simulink model "nn_ruido"  (R2023a)
settings: Solver=VariableStepAuto  StartTime=0.0  StopTime=1000  RelTol=1e-3
values from neighbouring files (symbols this model uses):
  A = 0.0154    [parametros.m]    (also in variables.mat)
  az1 = 1    [parametros.m]    (also in variables.mat)
  az2 = 1    [parametros.m]    (also in variables.mat)
  az3 = 1    [parametros.m]    (also in variables.mat)
  g = 9.8    [parametros.m]    (also in variables.mat)
  H_star1 = 0.4    [parametros.m]    (also in variables.mat)
  H_star2 = 0.15    [parametros.m]    (also in variables.mat)
  Sn = 5e-5    (= 5e-05)    [parametros.m]    (also in variables.mat)
settings Model: Creator=empg0  LastModifiedBy=empg0

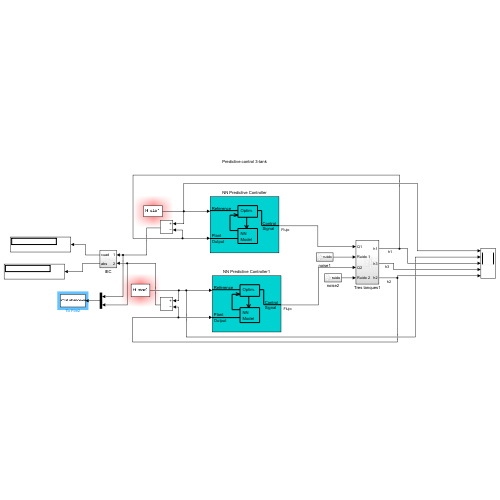
[thumbnail: Simulink's stored preview of the top-level diagram]
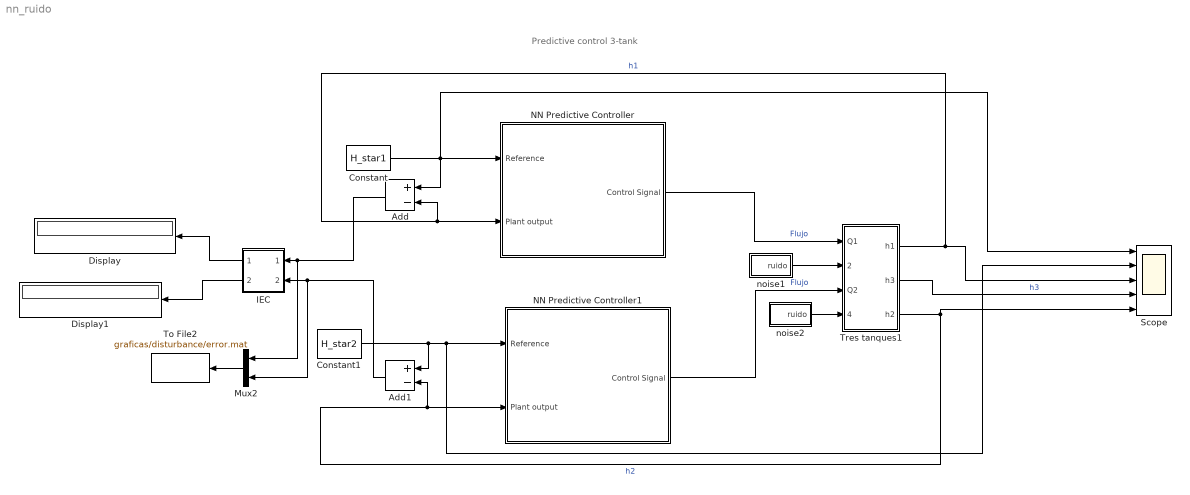
== system nn_ruido ==
  note: Predictive control 3-tank
  Add : Sum  Inputs=+-
  Add1 : Sum  Inputs=+-
  Constant : Constant  Value=H_star1
  Constant1 : Constant  Value=H_star2
  Display : Display
  Display1 : Display
  IEC : Subsystem
  Mux2 : Mux  Inputs=2
  NN Predictive Controller : Subsystem  mask(NN Predictive Controller){N2=7, Nu=2, Ts=0.5, rho=0.05, alpha=0.001, csrchfun=csrchbac, maxiter=2, S1=7, Ni=2, Nj=2, sim_file=planta, trainfun=trainlm, Use_validation=1, Use_Testing=0, max_i=0.1, min_i=0, sam_training=8000, epochs=200, minp=0.00083750919477898130849, maxp=0.099220790480832016245, mint=0, maxt=0.099220790480832016245, Normalize=0, IW=[-20.531676995171057598 18.704335179754611573;0.00020386653261894715898 -0.00065105597203892015979;0.11039206030581787121 0.078287285196172784474;-4.2899902912608469663 -2.5279624927180339711;-7.6432027343615454029 11.5285765668885265;-0.017993776662611957878 0.0088727669270464385592;-9.0344400995814524435 3.9540417662274571775], LW1_2=[14.923957143723018959 -17.978284009820111322;-0.71975082637667153751 0.32012412094941411489;0.64966823503412085561 0.085723391515673319496;55.495721009703864013 -51.282194417149113974;-3.6640121805562331225 2.3449172788885150887;-0.52558872900568831543 0.055226005018602114527;-1.7503201452350198863 4.144472061218764658], LW2_1=[-2.1959814678618032602 -3.2437397056361580994 7.2781964126742613175 2.1984051114526992343 1.7353616977917190045 -2.0712307468921604681 2.1983321974786087516], B1=[18.564420214207171256;9.6247423275479970783;-3.5269187756800972622;-67.658376524939384922;-4.4107470426168395861;0.061944283876979457093;-40.321949269656272463], B2=18.964938123059841502, max_i_int=20, min_i_int=5, limit_output=1, max_output=0.62, min_output=0, Use_Previous_Weights=1}
      mask prompts: Ts "Sample time"; rho "rho (typically = 0.03)"; alpha "alpha (typically = 0.001)"; csrchfun "Minimization rutine"; trainfun "Training function"
      mask help: NN Predictive Controller. You first train a neural network model of the plant to be controlled. The controller uses the plant model to predict plant performance over a specified time horizon. An optimization algorithm determines the control signal that optimizes plant performance over this horizon. Double click the NN Predictive Controller block to train the plant model and set the controller parameters.
      mask init:
      | xl = [0   .53   .53     .85   .85  .53  .53  NaN .85  .92 .92];
      | yl = [.95 .95 1.05  1.05   .82  .82  .95  NaN  .95 .95 .65];
      | x2 = [0 .53    NaN .92 1.2 NaN .53 .85 .85 .53 .53 ];
      | y2 = [.39 .39   NaN .65 .65 NaN .59 .59 .29 .29  .59];
      | x3 = [.67 .67 NaN .64 .67 .70 NaN .53 .4   .4   .53 NaN .46 .53 .46];
      | y3 = [.59 .82 NaN .66 .59 .66 NaN .55 .55 .86 .86 NaN  .89 .86 .83];
      | 
      | x1t=.03; y1t=.31;
      | x2t=.03; y2t=.8;
      | x8t=.03;y8t=.21;
      | x3t=.77; y3t=.53;
      | x4t=.77; y4t=.44;
      | x5t=.45; y5t=.76;
      | x6t=.45; y6t=.35;
      | x7t=.45; y7t=.25;
      settings: OpenFcn=nncontrolutil('nnpredict','',gcbh,gcb);
      mask TypeOptions csrchfun: csrchgol | csrchbac | csrchhyb | csrchbre | csrchcha
      mask TypeOptions trainfun: trainbfg | trainbr  | traincgb | traincgf | traincgp | traingd | traingdm | traingda | traingdx | trainlm  | trainoss | trainrp  | trainscg
      mask Display:
      | plot([[xl NaN x2]*.9-.075 ], [[yl  NaN y2]*.9-.1 ]);
      | plot([[x3]*.9-.075 ], [[y3]*.9-.1 ]);
      | text(x1t,y1t,'Plant');
      | text(x8t,y8t,'Output');
      | text(x2t,y2t,'Reference');
      | text(x3t,y3t,'Control');
      | text(x4t,y4t,'Signal');
      | text(x5t,y5t,'Optim.');
      | text(x6t,y6t,'NN');
      | text(x7t,y7t,'Model');
  NN Predictive Controller1 : Subsystem  mask(NN Predictive Controller){N2=7, Nu=2, Ts=0.5, rho=0.05, alpha=0.001, csrchfun=csrchbac, maxiter=2, S1=7, Ni=2, Nj=2, sim_file=planta, trainfun=trainlm, Use_validation=1, Use_Testing=0, max_i=0.1, min_i=0, sam_training=8000, epochs=200, minp=0.00083750919477898130849, maxp=0.099220790480832016245, mint=0, maxt=0.099220790480832016245, Normalize=0, IW=[-20.531676995171057598 18.704335179754611573;0.00020386653261894715898 -0.00065105597203892015979;0.11039206030581787121 0.078287285196172784474;-4.2899902912608469663 -2.5279624927180339711;-7.6432027343615454029 11.5285765668885265;-0.017993776662611957878 0.0088727669270464385592;-9.0344400995814524435 3.9540417662274571775], LW1_2=[14.923957143723018959 -17.978284009820111322;-0.71975082637667153751 0.32012412094941411489;0.64966823503412085561 0.085723391515673319496;55.495721009703864013 -51.282194417149113974;-3.6640121805562331225 2.3449172788885150887;-0.52558872900568831543 0.055226005018602114527;-1.7503201452350198863 4.144472061218764658], LW2_1=[-2.1959814678618032602 -3.2437397056361580994 7.2781964126742613175 2.1984051114526992343 1.7353616977917190045 -2.0712307468921604681 2.1983321974786087516], B1=[18.564420214207171256;9.6247423275479970783;-3.5269187756800972622;-67.658376524939384922;-4.4107470426168395861;0.061944283876979457093;-40.321949269656272463], B2=18.964938123059841502, max_i_int=20, min_i_int=5, limit_output=1, max_output=0.62, min_output=0, Use_Previous_Weights=1}
      mask prompts: Ts "Sample time"; rho "rho (typically = 0.03)"; alpha "alpha (typically = 0.001)"; csrchfun "Minimization rutine"; trainfun "Training function"
      mask help: NN Predictive Controller. You first train a neural network model of the plant to be controlled. The controller uses the plant model to predict plant performance over a specified time horizon. An optimization algorithm determines the control signal that optimizes plant performance over this horizon. Double click the NN Predictive Controller block to train the plant model and set the controller parameters.
      mask init: same as nn_ruido/NN Predictive Controller
      settings: OpenFcn=nncontrolutil('nnpredict','',gcbh,gcb);
      mask TypeOptions csrchfun: csrchgol | csrchbac | csrchhyb | csrchbre | csrchcha
      mask TypeOptions trainfun: trainbfg | trainbr  | traincgb | traincgf | traincgp | traingd | traingdm | traingda | traingdx | trainlm  | trainoss | trainrp  | trainscg
      mask Display:
      | plot([[xl NaN x2]*.9-.075 ], [[yl  NaN y2]*.9-.1 ]);
      | plot([[x3]*.9-.075 ], [[y3]*.9-.1 ]);
      | text(x1t,y1t,'Plant');
      | text(x8t,y8t,'Output');
      | text(x2t,y2t,'Reference');
      | text(x3t,y3t,'Control');
      | text(x4t,y4t,'Signal');
      | text(x5t,y5t,'Optim.');
      | text(x6t,y6t,'NN');
      | text(x7t,y7t,'Model');
  Scope : Scope  NumInputPorts=5
  To File2 : ToFile  Filename=graficas/disturbance/error.mat  MatrixName=error  SampleTime=0.5
  Tres tanques1 : Subsystem
  noise1 : Subsystem
  noise2 : Subsystem
  wires:
  NN Predictive Controller/1(Control Signal) -> Tres tanques1/1(Q1)  "Flujo"
  NN Predictive Controller1/1(Control Signal) -> Tres tanques1/3(Q2)  "Flujo"
  Tres tanques1/1(h1) -> Add/2, NN Predictive Controller/2(Plant output), Scope/3  "h1"
  Constant/1 -> Add/1, Scope/1, NN Predictive Controller/1(Reference)
  Constant1/1 -> Add1/1, Scope/2, NN Predictive Controller1/1(Reference)
  Tres tanques1/3(h2) -> Add1/2, NN Predictive Controller1/2(Plant output), Scope/5  "h2"
  Tres tanques1/2(h3) -> Scope/4  "h3"
  Add/1 -> Mux2/1, IEC/1(In1)
  Add1/1 -> Mux2/2, IEC/2(In2)
  IEC/1(cuad) -> Display/1
  Mux2/1 -> To File2/1
  noise1/1(ruido) -> Tres tanques1/2(Ruido 1)
  noise2/1(ruido) -> Tres tanques1/4(Ruido 2)
  IEC/2(abs) -> Display1/1

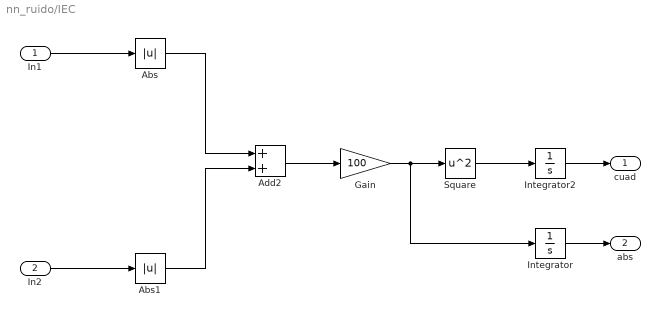
== system nn_ruido/IEC ==
  In1 : Inport
  In2 : Inport  Port=2
  Abs : Abs  SaturateOnIntegerOverflow=off
  Abs1 : Abs  SaturateOnIntegerOverflow=off
  Add2 : Sum
  Gain : Gain  Gain=100
  Integrator : Integrator
  Integrator2 : Integrator
  Square : Math  Operator=square
  cuad : Outport
  abs : Outport  Port=2
  wires:
  Abs1/1 -> Add2/2
  Abs/1 -> Add2/1
  In2/1 -> Abs1/1
  Square/1 -> Integrator2/1
  Integrator2/1 -> cuad/1
  In1/1 -> Abs/1
  Add2/1 -> Gain/1
  Gain/1 -> Integrator/1, Square/1
  Integrator/1 -> abs/1

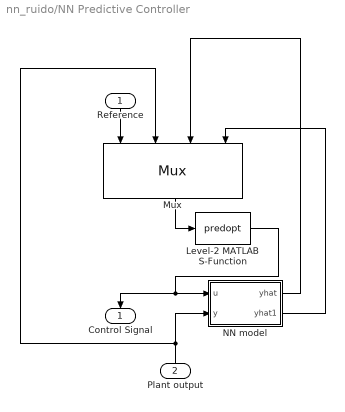
== system nn_ruido/NN Predictive Controller ==
  Reference : Inport
  Plant output : Inport  Port=2
  Level-2 MATLAB S-Function : M-S-Function  FunctionName=predopt  Parameters=N2,Ts,Nu,maxiter,csrchfun,rho,alpha,S1,IW,LW1_2,LW2_1,B1,B2,Ni,Nj,min_i,max_i,minp,maxp,mint,maxt,Normalize
  Mux : Mux
      settings: DisplayOption=signals
  NN model : Subsystem
  Control Signal : Outport
  wires:
  Mux/1 -> Level-2 MATLAB S-Function/1
  Level-2 MATLAB S-Function/1 -> NN model/1(u), Control Signal/1
  NN model/2(yhat1) -> Mux/4
  NN model/1(yhat) -> Mux/3
  Reference/1 -> Mux/1
  Plant output/1 -> NN model/2(y), Mux/2

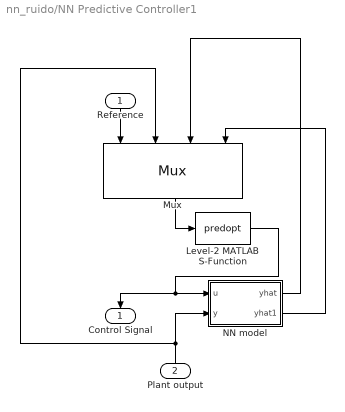
== system nn_ruido/NN Predictive Controller1 ==
  Reference : Inport
  Plant output : Inport  Port=2
  Level-2 MATLAB S-Function : M-S-Function  FunctionName=predopt  Parameters=N2,Ts,Nu,maxiter,csrchfun,rho,alpha,S1,IW,LW1_2,LW2_1,B1,B2,Ni,Nj,min_i,max_i,minp,maxp,mint,maxt,Normalize
  Mux : Mux
      settings: DisplayOption=signals
  NN model : Subsystem
  Control Signal : Outport
  wires:
  Mux/1 -> Level-2 MATLAB S-Function/1
  Level-2 MATLAB S-Function/1 -> NN model/1(u), Control Signal/1
  NN model/2(yhat1) -> Mux/4
  NN model/1(yhat) -> Mux/3
  Reference/1 -> Mux/1
  Plant output/1 -> NN model/2(y), Mux/2

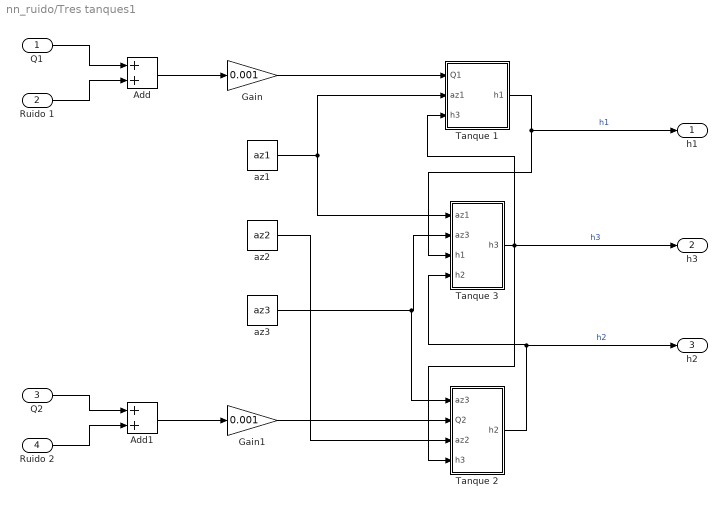
== system nn_ruido/Tres tanques1 ==
  Q1 : Inport
  Ruido 1 : Inport  Port=2
  Q2 : Inport  Port=3
  Ruido 2 : Inport  Port=4
  Add : Sum
  Add1 : Sum
  Gain : Gain  Gain=0.001
  Gain1 : Gain  Gain=0.001
  Tanque 1 : Subsystem
  Tanque 2 : Subsystem
  Tanque 3 : Subsystem
  az1 : Constant  Value=az1
  az2 : Constant  Value=az2
  az3 : Constant  Value=az3
  h1 : Outport
  h3 : Outport  Port=2
  h2 : Outport  Port=3
  wires:
  Tanque 2/1(h2) -> Tanque 3/4(h2), h2/1  "h2"
  Tanque 1/1(h1) -> Tanque 3/3(h1), h1/1  "h1"
  Gain1/1 -> Tanque 2/2(Q2)
  Tanque 3/1(h3) -> Tanque 2/4(h3), h3/1, Tanque 1/3(h3)  "h3"
  az3/1 -> Tanque 2/1(az3), Tanque 3/2(az3)
  az1/1 -> Tanque 3/1(az1), Tanque 1/2(az1)
  az2/1 -> Tanque 2/3(az2)
  Gain/1 -> Tanque 1/1(Q1)
  Add/1 -> Gain/1
  Q1/1 -> Add/1
  Ruido 1/1 -> Add/2
  Add1/1 -> Gain1/1
  Q2/1 -> Add1/1
  Ruido 2/1 -> Add1/2

== system nn_ruido/noise1 ==
  Constant : Constant  Value=0
  Manual Switch : ManualSwitch
  urn : UniformRandomNumber  Minimum=-0.1*0.1  Maximum=0.1*0.1  Seed=140  SampleTime=20
  ruido : Outport
  wires:
  urn/1 -> Manual Switch/1
  Constant/1 -> Manual Switch/2
  Manual Switch/1 -> ruido/1

== system nn_ruido/noise2 ==
  Constant : Constant  Value=0
  Manual Switch : ManualSwitch
  urn : UniformRandomNumber  Minimum=-0.1*0.1  Maximum=0.1*0.1  Seed=150  SampleTime=20
  ruido : Outport
  wires:
  urn/1 -> Manual Switch/1
  Constant/1 -> Manual Switch/2
  Manual Switch/1 -> ruido/1

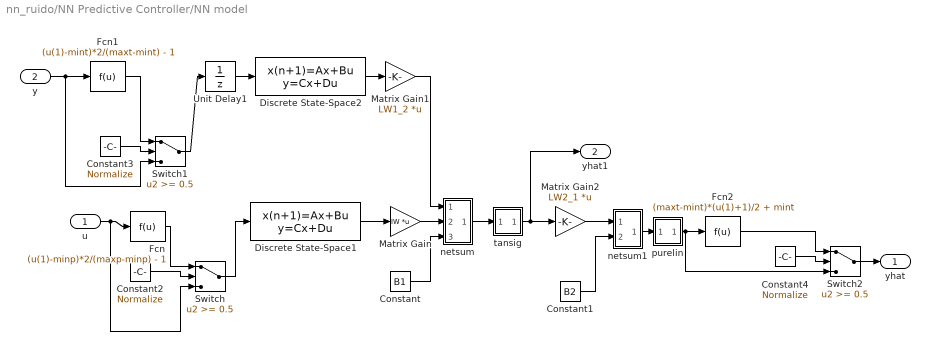
== system nn_ruido/NN Predictive Controller/NN model ==
  u : Inport
  y : Inport  Port=2
  Constant : Constant  Value=B1
  Constant1 : Constant  Value=B2
  Constant2 : Constant  Value=Normalize
  Constant3 : Constant  Value=Normalize
  Constant4 : Constant  Value=Normalize
  Discrete State-Space1 : DiscreteStateSpace  A=[0 zeros(1,Ni-2);eye(Ni-2,Ni-1)]  B=[zeros(double(Ni==1));eye(Ni-1,1)]  C=[0 zeros(1,Ni-2);eye(Ni-1,Ni-1)]  D=eye(Ni,1)  SampleTime=Ts
  Discrete State-Space2 : DiscreteStateSpace  A=[0 zeros(1,Nj-2);eye(Nj-2,Nj-1)]  B=[zeros(double(Nj==1));eye(Nj-1,1)]  C=[0 zeros(1,Nj-2);eye(Nj-1,Nj-1)]  D=eye(Nj,1)  SampleTime=Ts
  Fcn : Fcn  Expr=(u(1)-minp)*2/(maxp-minp) - 1
  Fcn1 : Fcn  Expr=(u(1)-mint)*2/(maxt-mint) - 1
  Fcn2 : Fcn  Expr=(maxt-mint)*(u(1)+1)/2 + mint
  Matrix Gain : Gain  Gain=IW  Multiplication=Matrix(K*u)  SaturateOnIntegerOverflow=on  OutDataTypeStr=Inherit: Same as input  ParamDataTypeStr=Inherit: Same as input
  Matrix Gain1 : Gain  Gain=LW1_2  Multiplication=Matrix(K*u)  SaturateOnIntegerOverflow=on  OutDataTypeStr=Inherit: Same as input  ParamDataTypeStr=Inherit: Same as input
  Matrix Gain2 : Gain  Gain=LW2_1  Multiplication=Matrix(K*u)  SaturateOnIntegerOverflow=on  OutDataTypeStr=Inherit: Same as input  ParamDataTypeStr=Inherit: Same as input
  Switch : Switch  Threshold=0.5  ZeroCross=off
  Switch1 : Switch  Threshold=0.5  ZeroCross=off
  Switch2 : Switch  Threshold=0.5  ZeroCross=off
  Unit Delay1 : UnitDelay  SampleTime=Ts  HasFrameUpgradeWarning=on
  netsum : Subsystem
      mask Display: disp('+')
  netsum1 : Subsystem
      mask Display: disp('+')
  purelin : Subsystem
      mask Display: plot([-1 1],[0 0],[-1 1],[-1 1])
  tansig : Subsystem
      mask Display: plot([-1 1],[0 0],[-1 -.9 -.8 -.7 -.6 -.5 -.4 -.3 -.2 -.1 0 .1 .2 .3 .4 .5 .6 .7 .8 .9 1],2./(1+exp(-8*[-1 -.9 -.8 -.7 -.6 -.5 -.4 -.3 -.2 -.1 0 .1 .2 .3 .4 .5 .6 .7 .8 .9 1]))-1)
  yhat : Outport
  yhat1 : Outport  Port=2
  wires:
  netsum1/1(Out1) -> purelin/1(n)
  Constant1/1 -> netsum1/2(In2)
  Matrix Gain2/1 -> netsum1/1(In1)
  netsum/1(Out1) -> tansig/1(n)
  Constant/1 -> netsum/3(In3)
  Matrix Gain1/1 -> netsum/1(In1)
  Matrix Gain/1 -> netsum/2(In2)
  tansig/1(a) -> Matrix Gain2/1, yhat1/1
  Discrete State-Space1/1 -> Matrix Gain/1
  Fcn/1 -> Switch/1
  Switch/1 -> Discrete State-Space1/1
  u/1 -> Fcn/1, Switch/3
  Constant2/1 -> Switch/2
  Discrete State-Space2/1 -> Matrix Gain1/1
  Unit Delay1/1 -> Discrete State-Space2/1
  Constant3/1 -> Switch1/2
  Switch1/1 -> Unit Delay1/1
  Fcn1/1 -> Switch1/1
  y/1 -> Fcn1/1, Switch1/3
  Constant4/1 -> Switch2/2
  Switch2/1 -> yhat/1
  Fcn2/1 -> Switch2/1
  purelin/1(a) -> Fcn2/1, Switch2/3

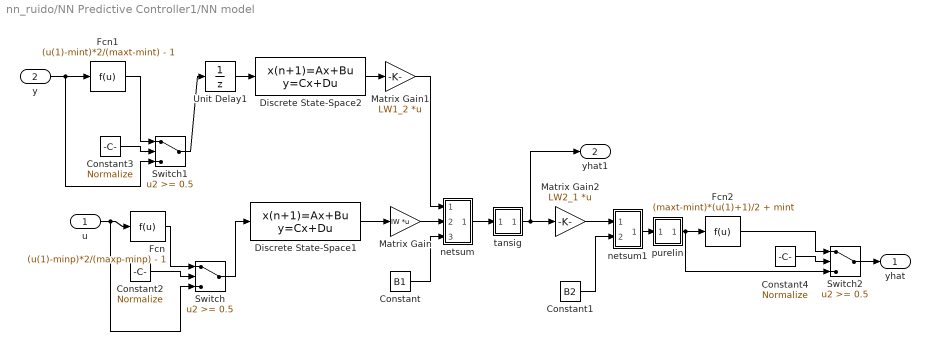
== system nn_ruido/NN Predictive Controller1/NN model ==
  u : Inport
  y : Inport  Port=2
  Constant : Constant  Value=B1
  Constant1 : Constant  Value=B2
  Constant2 : Constant  Value=Normalize
  Constant3 : Constant  Value=Normalize
  Constant4 : Constant  Value=Normalize
  Discrete State-Space1 : DiscreteStateSpace  A=[0 zeros(1,Ni-2);eye(Ni-2,Ni-1)]  B=[zeros(double(Ni==1));eye(Ni-1,1)]  C=[0 zeros(1,Ni-2);eye(Ni-1,Ni-1)]  D=eye(Ni,1)  SampleTime=Ts
  Discrete State-Space2 : DiscreteStateSpace  A=[0 zeros(1,Nj-2);eye(Nj-2,Nj-1)]  B=[zeros(double(Nj==1));eye(Nj-1,1)]  C=[0 zeros(1,Nj-2);eye(Nj-1,Nj-1)]  D=eye(Nj,1)  SampleTime=Ts
  Fcn : Fcn  Expr=(u(1)-minp)*2/(maxp-minp) - 1
  Fcn1 : Fcn  Expr=(u(1)-mint)*2/(maxt-mint) - 1
  Fcn2 : Fcn  Expr=(maxt-mint)*(u(1)+1)/2 + mint
  Matrix Gain : Gain  Gain=IW  Multiplication=Matrix(K*u)  SaturateOnIntegerOverflow=on  OutDataTypeStr=Inherit: Same as input  ParamDataTypeStr=Inherit: Same as input
  Matrix Gain1 : Gain  Gain=LW1_2  Multiplication=Matrix(K*u)  SaturateOnIntegerOverflow=on  OutDataTypeStr=Inherit: Same as input  ParamDataTypeStr=Inherit: Same as input
  Matrix Gain2 : Gain  Gain=LW2_1  Multiplication=Matrix(K*u)  SaturateOnIntegerOverflow=on  OutDataTypeStr=Inherit: Same as input  ParamDataTypeStr=Inherit: Same as input
  Switch : Switch  Threshold=0.5  ZeroCross=off
  Switch1 : Switch  Threshold=0.5  ZeroCross=off
  Switch2 : Switch  Threshold=0.5  ZeroCross=off
  Unit Delay1 : UnitDelay  SampleTime=Ts  HasFrameUpgradeWarning=on
  netsum : Subsystem
      mask Display: disp('+')
  netsum1 : Subsystem
      mask Display: disp('+')
  purelin : Subsystem
      mask Display: plot([-1 1],[0 0],[-1 1],[-1 1])
  tansig : Subsystem
      mask Display: plot([-1 1],[0 0],[-1 -.9 -.8 -.7 -.6 -.5 -.4 -.3 -.2 -.1 0 .1 .2 .3 .4 .5 .6 .7 .8 .9 1],2./(1+exp(-8*[-1 -.9 -.8 -.7 -.6 -.5 -.4 -.3 -.2 -.1 0 .1 .2 .3 .4 .5 .6 .7 .8 .9 1]))-1)
  yhat : Outport
  yhat1 : Outport  Port=2
  wires:
  netsum1/1(Out1) -> purelin/1(n)
  Constant1/1 -> netsum1/2(In2)
  Matrix Gain2/1 -> netsum1/1(In1)
  netsum/1(Out1) -> tansig/1(n)
  Constant/1 -> netsum/3(In3)
  Matrix Gain1/1 -> netsum/1(In1)
  Matrix Gain/1 -> netsum/2(In2)
  tansig/1(a) -> Matrix Gain2/1, yhat1/1
  Discrete State-Space1/1 -> Matrix Gain/1
  Fcn/1 -> Switch/1
  Switch/1 -> Discrete State-Space1/1
  u/1 -> Fcn/1, Switch/3
  Constant2/1 -> Switch/2
  Discrete State-Space2/1 -> Matrix Gain1/1
  Unit Delay1/1 -> Discrete State-Space2/1
  Constant3/1 -> Switch1/2
  Switch1/1 -> Unit Delay1/1
  Fcn1/1 -> Switch1/1
  y/1 -> Fcn1/1, Switch1/3
  Constant4/1 -> Switch2/2
  Switch2/1 -> yhat/1
  Fcn2/1 -> Switch2/1
  purelin/1(a) -> Fcn2/1, Switch2/3

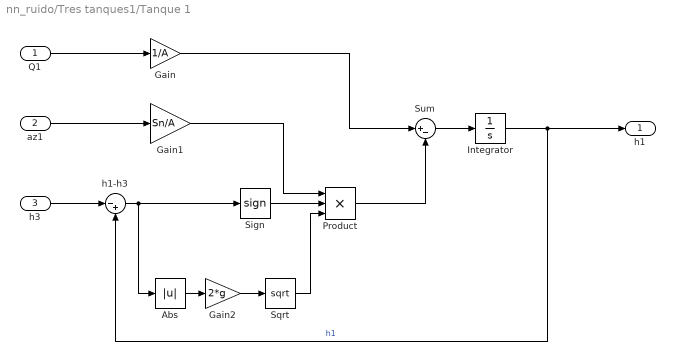
== system nn_ruido/Tres tanques1/Tanque 1 ==
  Q1 : Inport
  az1 : Inport  Port=2
  h3 : Inport  Port=3
  Abs : Abs  SaturateOnIntegerOverflow=off
  Gain : Gain  Gain=1/A
  Gain1 : Gain  Gain=Sn/A
  Gain2 : Gain  Gain=2*g
  Integrator : Integrator  LimitOutput=on  UpperSaturationLimit=0.62  LowerSaturationLimit=0
  Product : Product  Inputs=3
  Sign : Signum
  Sqrt : Sqrt
  Sum : Sum  Inputs=|+-
  h1-h3 : Sum  Inputs=|-+
  h1 : Outport
  wires:
  h3/1 -> h1-h3/1
  Sum/1 -> Integrator/1
  Gain2/1 -> Sqrt/1
  Gain1/1 -> Product/1
  Sqrt/1 -> Product/3
  Sign/1 -> Product/2
  h1-h3/1 -> Abs/1, Sign/1
  Q1/1 -> Gain/1
  az1/1 -> Gain1/1
  Integrator/1 -> h1/1, h1-h3/2  "h1"
  Product/1 -> Sum/2
  Gain/1 -> Sum/1
  Abs/1 -> Gain2/1

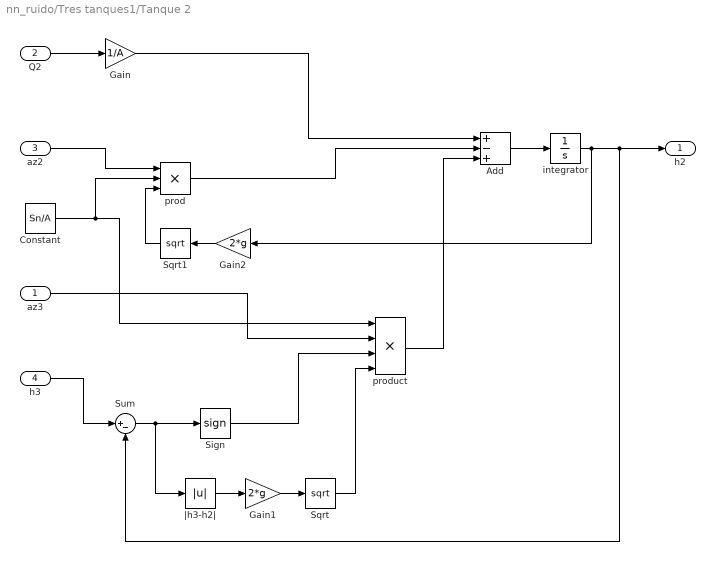
== system nn_ruido/Tres tanques1/Tanque 2 ==
  az3 : Inport
  Q2 : Inport  Port=2
  az2 : Inport  Port=3
  h3 : Inport  Port=4
  Add : Sum  Inputs=+-+
  Constant : Constant  Value=Sn/A
  Gain : Gain  Gain=1/A
  Gain1 : Gain  Gain=2*g
  Gain2 : Gain  Gain=2*g
  Sign : Signum
  Sqrt : Sqrt
  Sqrt1 : Sqrt
  Sum : Sum  Inputs=|+-
  integrator : Integrator  LimitOutput=on  UpperSaturationLimit=0.62  LowerSaturationLimit=0
  prod : Product  Inputs=3
  product : Product  Inputs=4
  |h3-h2| : Abs  SaturateOnIntegerOverflow=off
  h2 : Outport
  wires:
  |h3-h2|/1 -> Gain1/1
  prod/1 -> Add/2
  product/1 -> Add/3
  Add/1 -> integrator/1
  Gain/1 -> Add/1
  Constant/1 -> product/1, prod/2
  Gain1/1 -> Sqrt/1
  Sum/1 -> |h3-h2|/1, Sign/1
  az2/1 -> prod/1
  az3/1 -> product/2
  Sqrt1/1 -> prod/3
  Sqrt/1 -> product/4
  Sign/1 -> product/3
  h3/1 -> Sum/1
  integrator/1 -> Gain2/1, h2/1, Sum/2
  Gain2/1 -> Sqrt1/1
  Q2/1 -> Gain/1

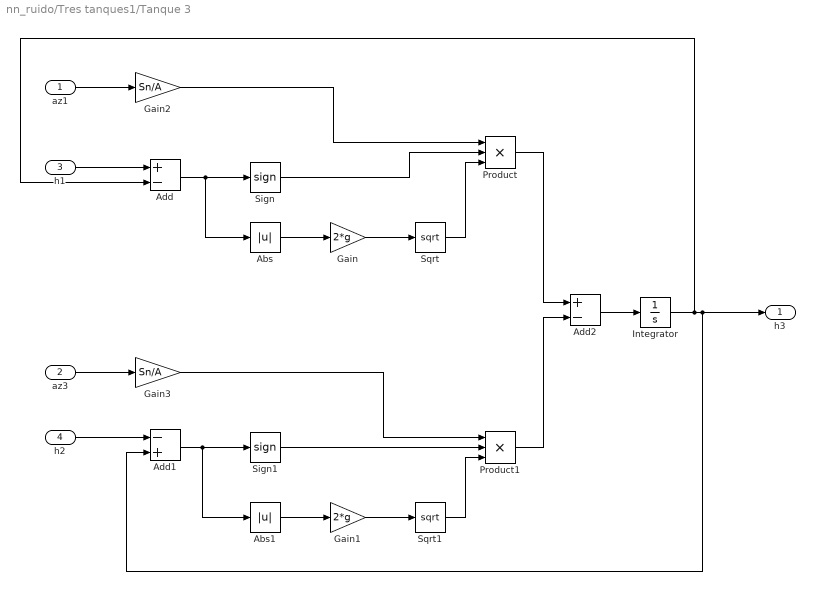
== system nn_ruido/Tres tanques1/Tanque 3 ==
  az1 : Inport
  az3 : Inport  Port=2
  h1 : Inport  Port=3
  h2 : Inport  Port=4
  Abs : Abs  SaturateOnIntegerOverflow=off
  Abs1 : Abs  SaturateOnIntegerOverflow=off
  Add : Sum  Inputs=+-
  Add1 : Sum  Inputs=-+
  Add2 : Sum  Inputs=+-
  Gain : Gain  Gain=2*g
  Gain1 : Gain  Gain=2*g
  Gain2 : Gain  Gain=Sn/A
  Gain3 : Gain  Gain=Sn/A
  Integrator : Integrator  LimitOutput=on  UpperSaturationLimit=0.62  LowerSaturationLimit=0
  Product : Product  Inputs=3
  Product1 : Product  Inputs=3
  Sign : Signum
  Sign1 : Signum
  Sqrt : Sqrt
  Sqrt1 : Sqrt
  h3 : Outport
  wires:
  Add2/1 -> Integrator/1
  Gain3/1 -> Product1/1
  az1/1 -> Gain2/1
  Gain1/1 -> Sqrt1/1
  Add1/1 -> Abs1/1, Sign1/1
  h1/1 -> Add/1
  az3/1 -> Gain3/1
  Integrator/1 -> h3/1, Add1/2, Add/2
  Abs1/1 -> Gain1/1
  Add/1 -> Abs/1, Sign/1
  Abs/1 -> Gain/1
  Sqrt1/1 -> Product1/3
  Sign/1 -> Product/2
  Product1/1 -> Add2/2
  Gain2/1 -> Product/1
  Sqrt/1 -> Product/3
  Sign1/1 -> Product1/2
  Gain/1 -> Sqrt/1
  h2/1 -> Add1/1
  Product/1 -> Add2/1

== system nn_ruido/NN Predictive Controller/NN model/netsum ==
  In1 : Inport
  In2 : Inport  Port=2
  In3 : Inport  Port=3
  netsum : Sum  Inputs=3  InputSameDT=on  SaturateOnIntegerOverflow=on  OutDataTypeStr=Inherit: Same as first input
  Out1 : Outport
  wires:
  In1/1 -> netsum/1
  In2/1 -> netsum/2
  In3/1 -> netsum/3
  netsum/1 -> Out1/1

== system nn_ruido/NN Predictive Controller/NN model/netsum1 ==
  In1 : Inport
  In2 : Inport  Port=2
  netsum1 : Sum  Inputs=2  InputSameDT=on  SaturateOnIntegerOverflow=on  OutDataTypeStr=Inherit: Same as first input
  Out1 : Outport
  wires:
  In1/1 -> netsum1/1
  In2/1 -> netsum1/2
  netsum1/1 -> Out1/1

== system nn_ruido/NN Predictive Controller/NN model/purelin ==
  n : Inport
  a : Outport
  wires:
  n/1 -> a/1

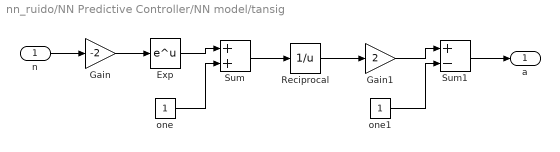
== system nn_ruido/NN Predictive Controller/NN model/tansig ==
  n : Inport
  Exp : Math  SignedPower=on
  Gain : Gain  Gain=-2  SaturateOnIntegerOverflow=on  OutDataTypeStr=Inherit: Same as input  ParamDataTypeStr=Inherit: Same as input
  Gain1 : Gain  Gain=2  SaturateOnIntegerOverflow=on  OutDataTypeStr=Inherit: Same as input  ParamDataTypeStr=Inherit: Same as input
  Reciprocal : Math  Operator=reciprocal  SignedPower=on
  Sum : Sum  InputSameDT=on  SaturateOnIntegerOverflow=on  OutDataTypeStr=Inherit: Same as first input
  Sum1 : Sum  Inputs=+-  InputSameDT=on  SaturateOnIntegerOverflow=on  OutDataTypeStr=Inherit: Same as first input
  one : Constant
  one1 : Constant
  a : Outport
  wires:
  n/1 -> Gain/1
  Gain/1 -> Exp/1
  Exp/1 -> Sum/1
  one/1 -> Sum/2
  Sum/1 -> Reciprocal/1
  Reciprocal/1 -> Gain1/1
  Gain1/1 -> Sum1/1
  one1/1 -> Sum1/2
  Sum1/1 -> a/1

== system nn_ruido/NN Predictive Controller1/NN model/netsum ==
  In1 : Inport
  In2 : Inport  Port=2
  In3 : Inport  Port=3
  netsum : Sum  Inputs=3  InputSameDT=on  SaturateOnIntegerOverflow=on  OutDataTypeStr=Inherit: Same as first input
  Out1 : Outport
  wires:
  In1/1 -> netsum/1
  In2/1 -> netsum/2
  In3/1 -> netsum/3
  netsum/1 -> Out1/1

== system nn_ruido/NN Predictive Controller1/NN model/netsum1 ==
  In1 : Inport
  In2 : Inport  Port=2
  netsum1 : Sum  Inputs=2  InputSameDT=on  SaturateOnIntegerOverflow=on  OutDataTypeStr=Inherit: Same as first input
  Out1 : Outport
  wires:
  In1/1 -> netsum1/1
  In2/1 -> netsum1/2
  netsum1/1 -> Out1/1

== system nn_ruido/NN Predictive Controller1/NN model/purelin ==
  n : Inport
  a : Outport
  wires:
  n/1 -> a/1

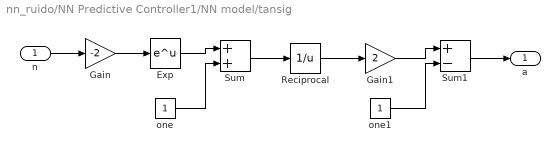
== system nn_ruido/NN Predictive Controller1/NN model/tansig ==
  n : Inport
  Exp : Math  SignedPower=on
  Gain : Gain  Gain=-2  SaturateOnIntegerOverflow=on  OutDataTypeStr=Inherit: Same as input  ParamDataTypeStr=Inherit: Same as input
  Gain1 : Gain  Gain=2  SaturateOnIntegerOverflow=on  OutDataTypeStr=Inherit: Same as input  ParamDataTypeStr=Inherit: Same as input
  Reciprocal : Math  Operator=reciprocal  SignedPower=on
  Sum : Sum  InputSameDT=on  SaturateOnIntegerOverflow=on  OutDataTypeStr=Inherit: Same as first input
  Sum1 : Sum  Inputs=+-  InputSameDT=on  SaturateOnIntegerOverflow=on  OutDataTypeStr=Inherit: Same as first input
  one : Constant
  one1 : Constant
  a : Outport
  wires:
  n/1 -> Gain/1
  Gain/1 -> Exp/1
  Exp/1 -> Sum/1
  one/1 -> Sum/2
  Sum/1 -> Reciprocal/1
  Reciprocal/1 -> Gain1/1
  Gain1/1 -> Sum1/1
  one1/1 -> Sum1/2
  Sum1/1 -> a/1
